simulink model "duplointegrador"  (R2020b)
settings: Solver=ode4  StartTime=0.0  StopTime=30  FixedStep=1e-3  RelTol=1e-3
undefined symbols (not defined in the file): Flqr, h, x10, x20
settings Model: Creator=Trevor  LastModifiedBy=lucas
settings SolverCC: AutoInsertRateTranBlk=on
settings DataIOCC: LimitDataPoints=on  SaveFormat=Array  ReturnWorkspaceOutputs=off
settings OptimizationCC: LifeSpan=inf
settings DebuggingCC: SFUnexpectedBacktrackingDiag=warning  SFNoUnconditionalDefaultTransitionDiag=warning  SFExecutionAtInitializationDiag=none  ArithmeticOperatorsInVariantConditions=warning
settings HardwareCC: ProdBitPerPointer=32  ProdBitPerSizeT=32  ProdBitPerPtrDiffT=32  ProdLargestAtomicFloat=None  ProdIntDivRoundTo=Undefined  ProdEndianess=Unspecified  ProdWordSize=32  ProdHWDeviceType=32-bit Generic
settings ModelReferenceCC: PropagateSignalLabelsOutOfModel=off
settings SFSimCC: SimUseLocalCustomCode=off  CustomCodeUndefinedFunction=UseInterfaceOnly
settings RTWCC: RTWUseLocalCustomCode=off
settings CodeAppCC: StateflowObjectComments=on
settings GRTTargetCC: TargetLangStandard=C89/C90 (ANSI)
settings ConfigComp: CovMetricSettings=dw  CovSaveCumulativeToWorkspaceVar=on  CovSaveSingleToWorkspaceVar=on  CovExternalEMLEnable=off

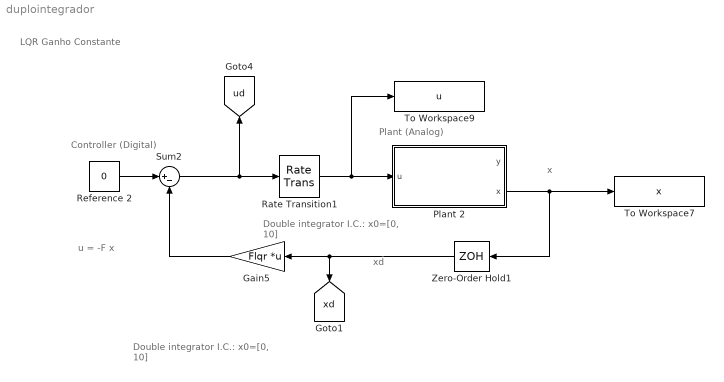
== system duplointegrador ==
  note: LQR Ganho Constante
  note: Double integrator
      | I.C.: x0=[0, 10]
  note: Controller (Digital)
  note: u = -F x
  note: xd
  note: x
  note: Plant (Analog)
  note: Double integrator
      | I.C.: x0=[0, 10]
  Gain5 : Gain  Gain=Flqr  Multiplication=Matrix(K*u)
  Plant 2 : Subsystem
      mask Display:
      | text(.5,.6,'dx/dt = Ax + Bu','horizontalAlignment', 'center','verticalAlignment', 'middle','texmode','on')
      | text(.5,.4,'y = Cx + Du','horizontalAlignment', 'center','verticalAlignment', 'middle','texmode','on')
      | port_label('input',1,'u')
      | port_label('output',1,'y')
      | port_label('output',2,'x')
  Rate Transition1 : RateTransition  Integrity=off  OutPortSampleTime=h
  Reference 2 : Constant  Value=0  SampleTime=h
  Sum2 : Sum  Inputs=|+-
  To Workspace7 : ToWorkspace  VariableName=x  SaveFormat=Timeseries  SampleTime=-1
  To Workspace9 : ToWorkspace  VariableName=u  SaveFormat=Timeseries  SampleTime=-1
  Zero-Order Hold1 : ZeroOrderHold  SampleTime=h
  tag scope: ud=global, xd=global
  wires:
  Sum2/1 -> Rate Transition1/1, [ud]
  Zero-Order Hold1/1 -> [xd], Gain5/1
  Gain5/1 -> Sum2/2
  Reference 2/1 -> Sum2/1
  Rate Transition1/1 -> Plant 2/1(u), To Workspace9/1
  Plant 2/2(x) -> To Workspace7/1, Zero-Order Hold1/1

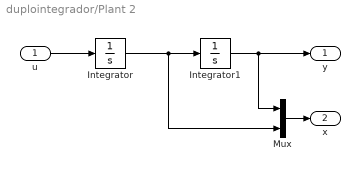
== system duplointegrador/Plant 2 ==
  u : Inport
  Integrator : Integrator  InitialCondition=x20
  Integrator1 : Integrator  InitialCondition=x10
  Mux : Mux  Inputs=2
  y : Outport
  x : Outport  Port=2
  wires:
  Integrator/1 -> Mux/2, Integrator1/1
  Integrator1/1 -> Mux/1, y/1
  u/1 -> Integrator/1
  Mux/1 -> x/1
